simulink model "SF006A_TEstimn"  (R2013b)
settings: Solver=FixedStepDiscrete  StartTime=0.0  StopTime=1  FixedStep=0.1  RelTol=1e-3
values from neighbouring files (symbols this model uses):
  ARCHGLBPRM_100MILLISEC_SEC_F32 = DataDict.Constant    [SF006A_TEstimn_DataDict.m]
  ARCHGLBPRM_2MILLISEC_SEC_F32 = DataDict.Constant    [SF006A_TEstimn_DataDict.m]
  TEstimnAmbPwrMplr = DataDict.Calibration    [SF006A_TEstimn_DataDict.m]
  TEstimnAmbTSca = DataDict.Calibration    [SF006A_TEstimn_DataDict.m]
  TEstimnAssiMechAmbMplr = DataDict.Calibration    [SF006A_TEstimn_DataDict.m]
  TEstimnAssiMechCorrLim = DataDict.Calibration    [SF006A_TEstimn_DataDict.m]
  TEstimnAssiMechDampgSca = DataDict.Calibration    [SF006A_TEstimn_DataDict.m]
  TEstimnAssiMechDftT = DataDict.Calibration    [SF006A_TEstimn_DataDict.m]
  TEstimnAssiMechLLFilCoeffA1 = DataDict.Calibration    [SF006A_TEstimn_DataDict.m]
  TEstimnAssiMechLLFilCoeffB0 = DataDict.Calibration    [SF006A_TEstimn_DataDict.m]
  TEstimnAssiMechLLFilCoeffB1 = DataDict.Calibration    [SF006A_TEstimn_DataDict.m]
  TEstimnAssiMechSlew = DataDict.Calibration    [SF006A_TEstimn_DataDict.m]
  TESTIMNASSIMECHTHILIM_DEGCGRD_F32 = DataDict.Constant    [SF006A_TEstimn_DataDict.m]
  TESTIMNASSIMECHTLOLIM_DEGCGRD_F32 = DataDict.Constant    [SF006A_TEstimn_DataDict.m]
  TEstimnCorrnTAssiMech = DataDict.Calibration    [SF006A_TEstimn_DataDict.m]
  TEstimnCorrnTCu = DataDict.Calibration    [SF006A_TEstimn_DataDict.m]
  TEstimnCorrnTMag = DataDict.Calibration    [SF006A_TEstimn_DataDict.m]
  TEstimnCorrnTSi = DataDict.Calibration    [SF006A_TEstimn_DataDict.m]
  TEstimnCuAmbMplr = DataDict.Calibration    [SF006A_TEstimn_DataDict.m]
  TEstimnCuCorrnLim = DataDict.Calibration    [SF006A_TEstimn_DataDict.m]
  TEstimnCuLLFilCoeffA1 = DataDict.Calibration    [SF006A_TEstimn_DataDict.m]
  TEstimnCuLLFilCoeffB0 = DataDict.Calibration    [SF006A_TEstimn_DataDict.m]
  TEstimnCuLLFilCoeffB1 = DataDict.Calibration    [SF006A_TEstimn_DataDict.m]
  TEstimnEngTSca = DataDict.Calibration    [SF006A_TEstimn_DataDict.m]
  TESTIMNFETTHILIM_DEGCGRD_F32 = DataDict.Constant    [SF006A_TEstimn_DataDict.m]
  TESTIMNFETTLOLIM_DEGCGRD_F32 = DataDict.Constant    [SF006A_TEstimn_DataDict.m]
  TEstimnMagAmbMplr = DataDict.Calibration    [SF006A_TEstimn_DataDict.m]
  TEstimnMagCorrnLim = DataDict.Calibration    [SF006A_TEstimn_DataDict.m]
  TEstimnMagLLFilCoeffA1 = DataDict.Calibration    [SF006A_TEstimn_DataDict.m]
  TEstimnMagLLFilCoeffB0 = DataDict.Calibration    [SF006A_TEstimn_DataDict.m]
  TEstimnMagLLFilCoeffB1 = DataDict.Calibration    [SF006A_TEstimn_DataDict.m]
  TESTIMNMAGTHILIM_DEGCGRD_F32 = DataDict.Constant    [SF006A_TEstimn_DataDict.m]
  TESTIMNMAGTLOLIM_DEGCGRD_F32 = DataDict.Constant    [SF006A_TEstimn_DataDict.m]
  TEstimnSiAmbMplr = DataDict.Calibration    [SF006A_TEstimn_DataDict.m]
  TEstimnSiCorrnLim = DataDict.Calibration    [SF006A_TEstimn_DataDict.m]
  TEstimnSiLLFilCoeffA1 = DataDict.Calibration    [SF006A_TEstimn_DataDict.m]
  TEstimnSiLLFilCoeffB0 = DataDict.Calibration    [SF006A_TEstimn_DataDict.m]
  TEstimnSiLLFilCoeffB1 = DataDict.Calibration    [SF006A_TEstimn_DataDict.m]
  TEstimnWghtAvrgTDi = DataDict.Calibration    [SF006A_TEstimn_DataDict.m]
  TESTIMNWIDGTHILIM_DEGCGRD_F32 = DataDict.Constant    [SF006A_TEstimn_DataDict.m]
  TESTIMNWIDGTLOLIM_DEGCGRD_F32 = DataDict.Constant    [SF006A_TEstimn_DataDict.m]
undefined symbols (not defined in the file or in its folder): sigbuilder_block
libraries: NxtrLim x13, Fil x8, simulink x2
(part 3 of 3)

== system SF006A_TEstimn/TEstimn/TEstimnPer1/TempEst/Lead//Lag Filter Function/Silicon Lead//Lag Filter ==
  note: When the Temperature Estimation function executes for the first time, the filter output
      | is set to CtrlTemp. The state variable will automatically be initialized.
      |
      | The initialization scheme can be mathematically expressed as follows,
      | y(0) = CtrlTemp;
      | x(0) = A1*y(0) + B1*u(0);
      | where y = output, x = state variable, u = input
      |
      | The general equation for the n-th time-step will be,
      | y(n) = x(n-1) + B0*u(n);
      | x(n) = A1*y(n-1) + B1*u(n-1);
      |
      | Note that if the filter output is initialized (to zero) when the value of CtrlTemp is not stable,
      | the state variable will get initialized to an incorrect value, and will result in grossly incorrect
      | temperature estimates.
      |
      | Note that the filter needs to be re-initialized using the specified method at the beginning of
      | each ignition cycle.
  EcuTFild : Inport
  Copyright1 : Subsystem  Description=|  RequirementInfo={} %GIDa_65003685_2a1c_45ef_ad34_5139a93f9eab  mask(Copyright Information){none=on}
      | Copyright info block.                                               
      |                                                                     
      | Place copyright information at the top of every subsystem in design.
      mask prompts: none "No parameters"
      mask help: Place copyright information at the top of every subsystem in design.
      mask Display:
      | NxtrConf = 'Nexteer Confidential';
      | 
      | sys = bdroot; %handle for the current model ("system")
      | first = get_param(sys,'Created');
      | if(isempty(first))
      |     first = datestr(now,'yyyy');
      | else
      |     first = first(end-3:end);  %year is last four digits
      | end
      | 
      | last = get_param(sys,'LastModifiedDate');
      | if isempty(last)
      |     last = datestr(now,'yyyy');
      | else
      |     last = last(end-3:end);
      | end
      | 
      | if strcmp(first,last)
      |     fprintf('%s\nCopyright  %s Nexteer',NxtrConf,first);
      | else
      |     fprintf('%s\n%s%s-%s Nexteer',NxtrConf,char(169),first,last);
      | end
  Data Store Read : DataStoreRead  DataStoreName=SiTEstimnPrev
  Data Store Write1 : DataStoreWrite  DataStoreName=SiTEstimnPrev
  Offset Copper Temperature : Constant  Value=TEstimnCorrnTSi
  Product (1) : Product  RndMeth=Zero
  Product (2) : Product  RndMeth=Zero
  Product (3) : Product  RndMeth=Zero
  Silicon Lead Lag Filter A1 : Constant  Value=TEstimnSiLLFilCoeffA1
  Silicon Lead Lag Filter B0 : Constant  Value=TEstimnSiLLFilCoeffB0
  Silicon Lead Lag Filter B1 : Constant  Value=TEstimnSiLLFilCoeffB1
  Sum (2)1 : Sum  Inputs=++|
  Sum (3)1 : Sum  Inputs=++|
  Sum (3)2 : Sum  Inputs=++|
  SiTempEst : Outport
  wires:
  Data Store Read/1 -> Sum (2)1/1
  Offset Copper Temperature/1 -> Sum (3)1/1
  Sum (3)1/1 -> Product (2)/2, Product (1)/2
  EcuTFild/1 -> Sum (3)1/2
  Sum (2)1/1 -> Product (3)/1, SiTempEst/1
  Silicon Lead Lag Filter A1/1 -> Product (3)/2
  Silicon Lead Lag Filter B1/1 -> Product (2)/1
  Product (2)/1 -> Sum (3)2/2
  Product (3)/1 -> Sum (3)2/1
  Silicon Lead Lag Filter B0/1 -> Product (1)/1
  Sum (3)2/1 -> Data Store Write1/1
  Product (1)/1 -> Sum (2)1/2

== system SF006A_TEstimn/TEstimn/TEstimnPer1/TempEst/Lead//Lag Filter Function/AssiMechTEstimnDisabled/Copyright1 ==

== system SF006A_TEstimn/TEstimn/TEstimnPer1/TempEst/Lead//Lag Filter Function/AssiMechTEstimnEnabled/Copyright1 ==

== system SF006A_TEstimn/TEstimn/TEstimnPer1/TempEst/Lead//Lag Filter Function/Assist Mechanism LeadLag Filter Initialization Periodic1/AssistMechanismInitDisable ==
  EcuTFild : Inport
  Action Port : ActionPort  ActionType=else
  Assist Mech Lead Lag Filter A2 : Constant  Value=TEstimnAssiMechLLFilCoeffA1
  Assist Mech Lead Lag Filter B1 : Constant  Value=TEstimnAssiMechLLFilCoeffB1
  Assist Mech Lead Lag Filter B2 : Constant  Value=TEstimnAssiMechLLFilCoeffB1
  Copyright1 : Subsystem  Description=|  RequirementInfo={} %GIDa_41ba1ae6_44a4_414c_9cc5_7c751333d8a8  mask(Copyright Information){none=on}
      | Copyright info block.                                               
      |                                                                     
      | Place copyright information at the top of every subsystem in design.
      mask prompts: none "No parameters"
      mask help: Place copyright information at the top of every subsystem in design.
      mask Display:
      | NxtrConf = 'Nexteer Confidential';
      | 
      | sys = bdroot; %handle for the current model ("system")
      | first = get_param(sys,'Created');
      | if(isempty(first))
      |     first = datestr(now,'yyyy');
      | else
      |     first = first(end-3:end);  %year is last four digits
      | end
      | 
      | last = get_param(sys,'LastModifiedDate');
      | if isempty(last)
      |     last = datestr(now,'yyyy');
      | else
      |     last = last(end-3:end);
      | end
      | 
      | if strcmp(first,last)
      |     fprintf('%s\nCopyright  %s Nexteer',NxtrConf,first);
      | else
      |     fprintf('%s\n%s%s-%s Nexteer',NxtrConf,char(169),first,last);
      | end
  Data Store Write1 : DataStoreWrite  DataStoreName=AssiMechTEstimnPrev
  Offset Assist Mech Temperature : Constant  Value=TEstimnCorrnTAssiMech
  Product (1)1 : Product  RndMeth=Zero
  Product (1)2 : Product  RndMeth=Zero
  Sum (2)2 : Sum  Inputs=++|
  Sum (4)1 : Sum  Inputs=+|+
  wires:
  Sum (4)1/1 -> Product (1)1/2
  Assist Mech Lead Lag Filter A2/1 -> Sum (4)1/1
  Assist Mech Lead Lag Filter B2/1 -> Sum (4)1/2
  Offset Assist Mech Temperature/1 -> Product (1)2/1
  Assist Mech Lead Lag Filter B1/1 -> Product (1)2/2
  Product (1)1/1 -> Sum (2)2/1
  Product (1)2/1 -> Sum (2)2/2
  Sum (2)2/1 -> Data Store Write1/1
  EcuTFild/1 -> Product (1)1/1

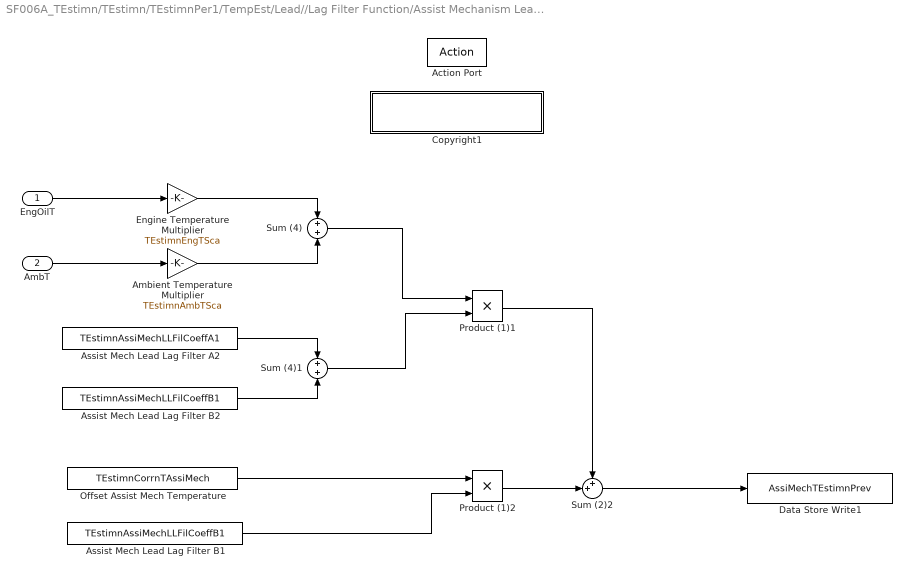
== system SF006A_TEstimn/TEstimn/TEstimnPer1/TempEst/Lead//Lag Filter Function/Assist Mechanism LeadLag Filter Initialization Periodic1/AssistMechanismInitEnable ==
  "EngOilT " : Inport
  AmbT : Inport  Port=2
  Action Port : ActionPort  ActionType=then
  Ambient Temperature Multiplier : Gain  Gain=TEstimnAmbTSca
      settings: AttributesFormatString=%<Gain>
  Assist Mech Lead Lag Filter A2 : Constant  Value=TEstimnAssiMechLLFilCoeffA1
  Assist Mech Lead Lag Filter B1 : Constant  Value=TEstimnAssiMechLLFilCoeffB1
  Assist Mech Lead Lag Filter B2 : Constant  Value=TEstimnAssiMechLLFilCoeffB1
  Copyright1 : Subsystem  Description=|  RequirementInfo={} %GIDa_198ddd45_1d5c_4f25_9681_a720f49e420b  mask(Copyright Information){none=on}
      | Copyright info block.                                               
      |                                                                     
      | Place copyright information at the top of every subsystem in design.
      mask prompts: none "No parameters"
      mask help: Place copyright information at the top of every subsystem in design.
      mask Display:
      | NxtrConf = 'Nexteer Confidential';
      | 
      | sys = bdroot; %handle for the current model ("system")
      | first = get_param(sys,'Created');
      | if(isempty(first))
      |     first = datestr(now,'yyyy');
      | else
      |     first = first(end-3:end);  %year is last four digits
      | end
      | 
      | last = get_param(sys,'LastModifiedDate');
      | if isempty(last)
      |     last = datestr(now,'yyyy');
      | else
      |     last = last(end-3:end);
      | end
      | 
      | if strcmp(first,last)
      |     fprintf('%s\nCopyright  %s Nexteer',NxtrConf,first);
      | else
      |     fprintf('%s\n%s%s-%s Nexteer',NxtrConf,char(169),first,last);
      | end
  Data Store Write1 : DataStoreWrite  DataStoreName=AssiMechTEstimnPrev
  Engine Temperature Multiplier : Gain  Gain=TEstimnEngTSca
      settings: AttributesFormatString=%<Gain>
  Offset Assist Mech Temperature : Constant  Value=TEstimnCorrnTAssiMech
  Product (1)1 : Product  RndMeth=Zero
  Product (1)2 : Product  RndMeth=Zero
  Sum (2)2 : Sum  Inputs=++|
  Sum (4) : Sum  Inputs=+|+
  Sum (4)1 : Sum  Inputs=+|+
  wires:
  "EngOilT "/1 -> Engine Temperature Multiplier/1
  Engine Temperature Multiplier/1 -> Sum (4)/1
  Ambient Temperature Multiplier/1 -> Sum (4)/2
  AmbT/1 -> Ambient Temperature Multiplier/1
  Sum (4)/1 -> Product (1)1/1
  Sum (4)1/1 -> Product (1)1/2
  Assist Mech Lead Lag Filter A2/1 -> Sum (4)1/1
  Assist Mech Lead Lag Filter B2/1 -> Sum (4)1/2
  Offset Assist Mech Temperature/1 -> Product (1)2/1
  Assist Mech Lead Lag Filter B1/1 -> Product (1)2/2
  Product (1)1/1 -> Sum (2)2/1
  Product (1)2/1 -> Sum (2)2/2
  Sum (2)2/1 -> Data Store Write1/1

== system SF006A_TEstimn/TEstimn/TEstimnPer1/TempEst/Lead//Lag Filter Function/Assist Mechanism LeadLag Filter Initialization Periodic1/Copyright1 ==

== system SF006A_TEstimn/TEstimn/TEstimnPer1/TempEst/Lead//Lag Filter Function/AssistMechanism Lead//Lag Filter/AssiMechTCalcnDisabled ==
  WtAvgTemp : Inport
  Action Port : ActionPort  ActionType=then
  Copyright1 : Subsystem  Description=|  RequirementInfo={} %GIDa_5edaeb55_7c1a_4591_a888_51e88ae00594  mask(Copyright Information){none=on}
      | Copyright info block.                                               
      |                                                                     
      | Place copyright information at the top of every subsystem in design.
      mask prompts: none "No parameters"
      mask help: Place copyright information at the top of every subsystem in design.
      mask Display:
      | NxtrConf = 'Nexteer Confidential';
      | 
      | sys = bdroot; %handle for the current model ("system")
      | first = get_param(sys,'Created');
      | if(isempty(first))
      |     first = datestr(now,'yyyy');
      | else
      |     first = first(end-3:end);  %year is last four digits
      | end
      | 
      | last = get_param(sys,'LastModifiedDate');
      | if isempty(last)
      |     last = datestr(now,'yyyy');
      | else
      |     last = last(end-3:end);
      | end
      | 
      | if strcmp(first,last)
      |     fprintf('%s\nCopyright  %s Nexteer',NxtrConf,first);
      | else
      |     fprintf('%s\n%s%s-%s Nexteer',NxtrConf,char(169),first,last);
      | end
  Offset Assist Mech Temperature : Constant  Value=TEstimnCorrnTAssiMech
  Sum (3)1 : Sum  Inputs=++|
  AssiMechTCalcn : Outport
  wires:
  Offset Assist Mech Temperature/1 -> Sum (3)1/1
  WtAvgTemp/1 -> Sum (3)1/2
  Sum (3)1/1 -> AssiMechTCalcn/1

== system SF006A_TEstimn/TEstimn/TEstimnPer1/TempEst/Lead//Lag Filter Function/AssistMechanism Lead//Lag Filter/AssiMechTCalcnEnabled ==
  EcuTFild : Inport
  Action Port : ActionPort  ActionType=else
  Copyright1 : Subsystem  Description=|  RequirementInfo={} %GIDa_ef3e647a_f4bd_40b1_8bad_ddabf82cc225  mask(Copyright Information){none=on}
      | Copyright info block.                                               
      |                                                                     
      | Place copyright information at the top of every subsystem in design.
      mask prompts: none "No parameters"
      mask help: Place copyright information at the top of every subsystem in design.
      mask Display:
      | NxtrConf = 'Nexteer Confidential';
      | 
      | sys = bdroot; %handle for the current model ("system")
      | first = get_param(sys,'Created');
      | if(isempty(first))
      |     first = datestr(now,'yyyy');
      | else
      |     first = first(end-3:end);  %year is last four digits
      | end
      | 
      | last = get_param(sys,'LastModifiedDate');
      | if isempty(last)
      |     last = datestr(now,'yyyy');
      | else
      |     last = last(end-3:end);
      | end
      | 
      | if strcmp(first,last)
      |     fprintf('%s\nCopyright  %s Nexteer',NxtrConf,first);
      | else
      |     fprintf('%s\n%s%s-%s Nexteer',NxtrConf,char(169),first,last);
      | end
  Offset Assist Mech Temperature : Constant  Value=TEstimnCorrnTAssiMech
  Sum (3)1 : Sum  Inputs=++|
  "AssiMechTCalcn " : Outport
  wires:
  Offset Assist Mech Temperature/1 -> Sum (3)1/1
  Sum (3)1/1 -> "AssiMechTCalcn "/1
  EcuTFild/1 -> Sum (3)1/2

== system SF006A_TEstimn/TEstimn/TEstimnPer1/TempEst/Lead//Lag Filter Function/AssistMechanism Lead//Lag Filter/Copyright1 ==

== system SF006A_TEstimn/TEstimn/TEstimnPer1/TempEst/Lead//Lag Filter Function/AssistMechanism Lead//Lag Filter/PreAssiMechTEstimEnabled ==
  "AssiMechTCalcn " : Inport
  Assist Mech Lead Lag Filter A1 : Constant  Value=TEstimnAssiMechLLFilCoeffA1
  Assist Mech Lead Lag Filter B0 : Constant  Value=TEstimnAssiMechLLFilCoeffB0
  Assist Mech Lead Lag Filter B1 : Constant  Value=TEstimnAssiMechLLFilCoeffB1
  Copyright1 : Subsystem  Description=|  RequirementInfo={} %GIDa_9c2fd809_04d8_4a50_8cde_9595a1867e4b  mask(Copyright Information){none=on}
      | Copyright info block.                                               
      |                                                                     
      | Place copyright information at the top of every subsystem in design.
      mask prompts: none "No parameters"
      mask help: Place copyright information at the top of every subsystem in design.
      mask Display:
      | NxtrConf = 'Nexteer Confidential';
      | 
      | sys = bdroot; %handle for the current model ("system")
      | first = get_param(sys,'Created');
      | if(isempty(first))
      |     first = datestr(now,'yyyy');
      | else
      |     first = first(end-3:end);  %year is last four digits
      | end
      | 
      | last = get_param(sys,'LastModifiedDate');
      | if isempty(last)
      |     last = datestr(now,'yyyy');
      | else
      |     last = last(end-3:end);
      | end
      | 
      | if strcmp(first,last)
      |     fprintf('%s\nCopyright  %s Nexteer',NxtrConf,first);
      | else
      |     fprintf('%s\n%s%s-%s Nexteer',NxtrConf,char(169),first,last);
      | end
  Data Store Write2 : DataStoreWrite  DataStoreName=AssiMechTEstimnPrev
  PreAssiMechTEstimn_FB : DataStoreRead  DataStoreName=AssiMechTEstimnPrev
  Product (1)1 : Product  RndMeth=Zero
  Product (2) : Product  RndMeth=Zero
  Product (3) : Product  RndMeth=Zero
  Sum (2)1 : Sum  Inputs=++|
  Sum (3)4 : Sum  Inputs=++|
  AssiMechTEstimn : Outport
  wires:
  PreAssiMechTEstimn_FB/1 -> Sum (2)1/1
  "AssiMechTCalcn "/1 -> Product (2)/2, Product (1)1/2
  Sum (2)1/1 -> AssiMechTEstimn/1, Product (3)/1
  Assist Mech Lead Lag Filter A1/1 -> Product (3)/2
  Assist Mech Lead Lag Filter B1/1 -> Product (2)/1
  Product (2)/1 -> Sum (3)4/2
  Product (3)/1 -> Sum (3)4/1
  Assist Mech Lead Lag Filter B0/1 -> Product (1)1/1
  Sum (3)4/1 -> Data Store Write2/1
  Product (1)1/1 -> Sum (2)1/2

== system SF006A_TEstimn/TEstimn/TEstimnPer1/TempEst/Lead//Lag Filter Function/AssistMechanismLeadLagFilterRe-Initialization/AssistMechanismInitDisable ==
  EcuTFild : Inport
  Action Port : ActionPort  ActionType=else
  Assist Mech Lead Lag Filter A2 : Constant  Value=TEstimnAssiMechLLFilCoeffA1
  Assist Mech Lead Lag Filter B1 : Constant  Value=TEstimnAssiMechLLFilCoeffB1
  Assist Mech Lead Lag Filter B2 : Constant  Value=TEstimnAssiMechLLFilCoeffB1
  Copyright1 : Subsystem  Description=|  RequirementInfo={} %GIDa_dbe726fd_0257_4e1b_be64_24b37b0faac1  mask(Copyright Information){none=on}
      | Copyright info block.                                               
      |                                                                     
      | Place copyright information at the top of every subsystem in design.
      mask prompts: none "No parameters"
      mask help: Place copyright information at the top of every subsystem in design.
      mask Display:
      | NxtrConf = 'Nexteer Confidential';
      | 
      | sys = bdroot; %handle for the current model ("system")
      | first = get_param(sys,'Created');
      | if(isempty(first))
      |     first = datestr(now,'yyyy');
      | else
      |     first = first(end-3:end);  %year is last four digits
      | end
      | 
      | last = get_param(sys,'LastModifiedDate');
      | if isempty(last)
      |     last = datestr(now,'yyyy');
      | else
      |     last = last(end-3:end);
      | end
      | 
      | if strcmp(first,last)
      |     fprintf('%s\nCopyright  %s Nexteer',NxtrConf,first);
      | else
      |     fprintf('%s\n%s%s-%s Nexteer',NxtrConf,char(169),first,last);
      | end
  Data Store Write1 : DataStoreWrite  DataStoreName=AssiMechTEstimnPrev
  Offset Assist Mech Temperature : Constant  Value=TEstimnCorrnTAssiMech
  Product (1)1 : Product  RndMeth=Zero
  Product (1)2 : Product  RndMeth=Zero
  Sum (2)2 : Sum  Inputs=++|
  Sum (4)1 : Sum  Inputs=+|+
  wires:
  Sum (4)1/1 -> Product (1)1/2
  Assist Mech Lead Lag Filter A2/1 -> Sum (4)1/1
  Assist Mech Lead Lag Filter B2/1 -> Sum (4)1/2
  Offset Assist Mech Temperature/1 -> Product (1)2/1
  Assist Mech Lead Lag Filter B1/1 -> Product (1)2/2
  Product (1)1/1 -> Sum (2)2/1
  Product (1)2/1 -> Sum (2)2/2
  Sum (2)2/1 -> Data Store Write1/1
  EcuTFild/1 -> Product (1)1/1

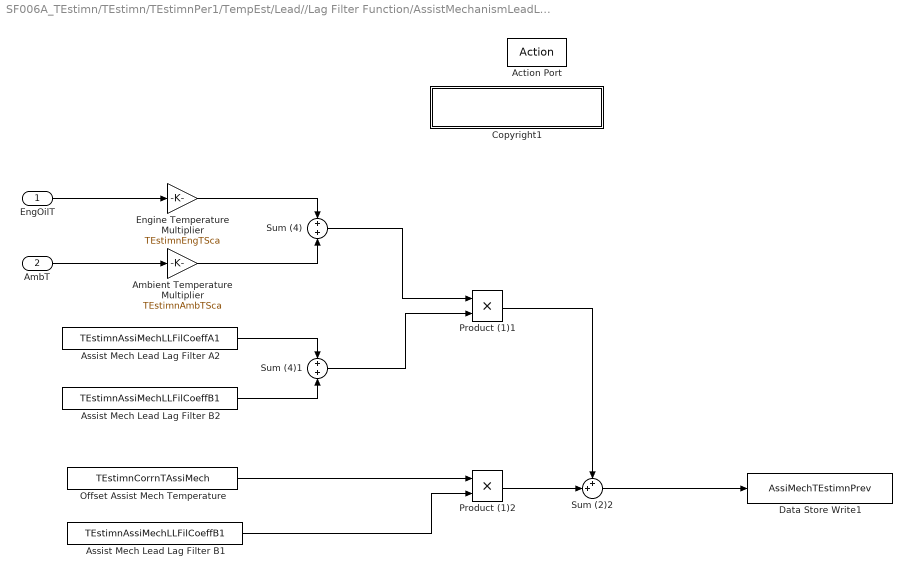
== system SF006A_TEstimn/TEstimn/TEstimnPer1/TempEst/Lead//Lag Filter Function/AssistMechanismLeadLagFilterRe-Initialization/AssistMechanismInitEnable ==
  "EngOilT " : Inport
  AmbT : Inport  Port=2
  Action Port : ActionPort  ActionType=then
  Ambient Temperature Multiplier : Gain  Gain=TEstimnAmbTSca
      settings: AttributesFormatString=%<Gain>
  Assist Mech Lead Lag Filter A2 : Constant  Value=TEstimnAssiMechLLFilCoeffA1
  Assist Mech Lead Lag Filter B1 : Constant  Value=TEstimnAssiMechLLFilCoeffB1
  Assist Mech Lead Lag Filter B2 : Constant  Value=TEstimnAssiMechLLFilCoeffB1
  Copyright1 : Subsystem  Description=|  RequirementInfo={} %GIDa_c077be1b_432a_4f6c_a5a9_63c891af496e  mask(Copyright Information){none=on}
      | Copyright info block.                                               
      |                                                                     
      | Place copyright information at the top of every subsystem in design.
      mask prompts: none "No parameters"
      mask help: Place copyright information at the top of every subsystem in design.
      mask Display:
      | NxtrConf = 'Nexteer Confidential';
      | 
      | sys = bdroot; %handle for the current model ("system")
      | first = get_param(sys,'Created');
      | if(isempty(first))
      |     first = datestr(now,'yyyy');
      | else
      |     first = first(end-3:end);  %year is last four digits
      | end
      | 
      | last = get_param(sys,'LastModifiedDate');
      | if isempty(last)
      |     last = datestr(now,'yyyy');
      | else
      |     last = last(end-3:end);
      | end
      | 
      | if strcmp(first,last)
      |     fprintf('%s\nCopyright  %s Nexteer',NxtrConf,first);
      | else
      |     fprintf('%s\n%s%s-%s Nexteer',NxtrConf,char(169),first,last);
      | end
  Data Store Write1 : DataStoreWrite  DataStoreName=AssiMechTEstimnPrev
  Engine Temperature Multiplier : Gain  Gain=TEstimnEngTSca
      settings: AttributesFormatString=%<Gain>
  Offset Assist Mech Temperature : Constant  Value=TEstimnCorrnTAssiMech
  Product (1)1 : Product  RndMeth=Zero
  Product (1)2 : Product  RndMeth=Zero
  Sum (2)2 : Sum  Inputs=++|
  Sum (4) : Sum  Inputs=+|+
  Sum (4)1 : Sum  Inputs=+|+
  wires:
  "EngOilT "/1 -> Engine Temperature Multiplier/1
  Engine Temperature Multiplier/1 -> Sum (4)/1
  Ambient Temperature Multiplier/1 -> Sum (4)/2
  AmbT/1 -> Ambient Temperature Multiplier/1
  Sum (4)/1 -> Product (1)1/1
  Sum (4)1/1 -> Product (1)1/2
  Assist Mech Lead Lag Filter A2/1 -> Sum (4)1/1
  Assist Mech Lead Lag Filter B2/1 -> Sum (4)1/2
  Offset Assist Mech Temperature/1 -> Product (1)2/1
  Assist Mech Lead Lag Filter B1/1 -> Product (1)2/2
  Product (1)1/1 -> Sum (2)2/1
  Product (1)2/1 -> Sum (2)2/2
  Sum (2)2/1 -> Data Store Write1/1

== system SF006A_TEstimn/TEstimn/TEstimnPer1/TempEst/Lead//Lag Filter Function/AssistMechanismLeadLagFilterRe-Initialization/Copyright1 ==

== system SF006A_TEstimn/TEstimn/TEstimnPer1/TempEst/Lead//Lag Filter Function/Copper Lead//Lag Filter/Copyright1 ==

== system SF006A_TEstimn/TEstimn/TEstimnPer1/TempEst/Lead//Lag Filter Function/Magnet Lead//Lag Filter/Copyright1 ==

== system SF006A_TEstimn/TEstimn/TEstimnPer1/TempEst/Lead//Lag Filter Function/Silicon Lead//Lag Filter/Copyright1 ==

== system SF006A_TEstimn/TEstimn/TEstimnPer1/TempEst/Lead//Lag Filter Function/Assist Mechanism LeadLag Filter Initialization Periodic1/AssistMechanismInitDisable/Copyright1 ==

== system SF006A_TEstimn/TEstimn/TEstimnPer1/TempEst/Lead//Lag Filter Function/Assist Mechanism LeadLag Filter Initialization Periodic1/AssistMechanismInitEnable/Copyright1 ==

== system SF006A_TEstimn/TEstimn/TEstimnPer1/TempEst/Lead//Lag Filter Function/AssistMechanism Lead//Lag Filter/AssiMechTCalcnDisabled/Copyright1 ==

== system SF006A_TEstimn/TEstimn/TEstimnPer1/TempEst/Lead//Lag Filter Function/AssistMechanism Lead//Lag Filter/AssiMechTCalcnEnabled/Copyright1 ==

== system SF006A_TEstimn/TEstimn/TEstimnPer1/TempEst/Lead//Lag Filter Function/AssistMechanism Lead//Lag Filter/PreAssiMechTEstimEnabled/Copyright1 ==

== system SF006A_TEstimn/TEstimn/TEstimnPer1/TempEst/Lead//Lag Filter Function/AssistMechanismLeadLagFilterRe-Initialization/AssistMechanismInitDisable/Copyright1 ==

== system SF006A_TEstimn/TEstimn/TEstimnPer1/TempEst/Lead//Lag Filter Function/AssistMechanismLeadLagFilterRe-Initialization/AssistMechanismInitEnable/Copyright1 ==
